simulink model "milemate_digital_twin"  (R2026a)
settings: Solver=VariableStepAuto  StopTime=500  MaxStep=0.05
libraries: sim3dlib x36
(part 4 of 5)

== matlab function milemate_digital_twin/MATLAB Function ==
  data: floor1_visual_id input size=[5 1]; floor1_visible input size=[50 1]; floor1_color_flag input size=[50 1]; platform_y input size=[1 1]; floor1_visual_count input size=[1 1]; pkg1_T output; pkg2_T output; pkg3_T output; pkg4_T output; pkg5_T output; pkg1_R output; pkg2_R output; pkg3_R output; pkg4_R output; pkg5_R output; pkg1_S output; pkg2_S output; pkg3_S output; pkg4_S output; pkg5_S output; target_unload_id input size=[1 1]; highlight_enable input size=[1 1]; target_package_on_belt4 input size=[1 1]; package_on_platform_from_floor input; platform_z input; current_unload_id input; floor1_visual_path input size=[5 1]; target_list input size=[20 1]; target_count input size=[1 1]; pkg1_Color output; pkg2_Color output; pkg3_Color output; pkg4_Color output; pkg5_Color output; belt4_reverse_progress input size=[1 1]; belt4_reverse_phase input size=[1 1]
function [pkg1_T, pkg2_T, pkg3_T, pkg4_T, pkg5_T, ...
          pkg1_R, pkg2_R, pkg3_R, pkg4_R, pkg5_R, ...
          pkg1_S, pkg2_S, pkg3_S, pkg4_S, pkg5_S, ...
          pkg1_Color, pkg2_Color, pkg3_Color, pkg4_Color, pkg5_Color] = ...
          Package3DMappingFunction_F1(floor1_visual_id, floor1_visible, floor1_color_flag, platform_y, floor1_visual_count, ...
                                      target_unload_id, highlight_enable, target_package_on_belt4, ...
                                      package_on_platform_from_floor, platform_z, current_unload_id, floor1_visual_path, ...
                                      target_list, target_count, belt4_reverse_progress, belt4_reverse_phase)
% Package3DMappingFunction_F1
% 1층 정적/연속 이동 박스 표시 함수
%
% 중요:
% - 이제 F1은 FloorStorageUpdate/floor1_queue 또는 PackageSlotVisualizer/floor1_slot_id를 직접 쓰지 않는다.
% - Floor1VisualStateFunction이 저장한 floor1_visual_id, floor1_visual_path를 기준으로 표시한다.
% - visual_shift는 이 함수에 직접 들어오지 않는다.
%
% 입력:
% floor1_visual_id               [5x1]
% floor1_visible                 [50x1]  % 기존 포트 유지용
% floor1_color_flag              [50x1]  % 기존 포트 유지용
% platform_y                     [1x1]
% floor1_visual_count            [1x1]
% target_unload_id               [1x1]  % 1층 하차공간 준비 대상
% highlight_enable               [1x1]
% target_package_on_belt4        [1x1]
% package_on_platform_from_floor [1x1]
% platform_z                     [1x1]
% current_unload_id              [1x1]  % 현재 실제 하차 대상
% floor1_visual_path             [5x1]

% =========================
% 박스 크기
% =========================
pkg_short = 0.12;
pkg_long  = 0.16;
pkg_h     = 0.08;

pkg_scale = [pkg_short, pkg_long, pkg_h];

% =========================
% 색상 설정
% =========================
normal_color = [0.75, 0.45, 0.20];
target_color = [1.0, 1.0, 0.0];

% =========================
% 1층 높이
% =========================
z_floor1 = 0.00;
pkg_center_z = z_floor1 + pkg_h / 2;

hide_z = -10.0;

% =========================
% 컨베이어 기준값
% =========================
belt_width = 0.25;

L1 = 0.51;
L3 = 0.51;
L4 = 1.11;

stopper_x = -0.15;
stopper_y = platform_y + 0.30;
stopper_thick_x = 0.03;

A_x = stopper_x - stopper_thick_x / 2;
A_y = stopper_y;

side_y = 1;
side_x = 1;

% =========================
% Belt3 geometry
% =========================
belt3_right_x = A_x;
belt3_center_y = A_y;
belt3_connect_edge_y = belt3_center_y + side_y * belt_width / 2;

% =========================
% Belt4 geometry
% =========================
if side_x > 0
    belt4_left_x  = A_x;
    belt4_right_x = A_x + belt_width;
else
    belt4_left_x  = A_x - belt_width;
    belt4_right_x = A_x;
end

belt4_center_x = (belt4_left_x + belt4_right_x) / 2;

belt4_start_y_nominal = belt3_connect_edge_y;
belt4_platform_extend = 0.25;

belt4_start_y = belt4_start_y_nominal - side_y * belt4_platform_extend;
belt4_end_y = belt4_start_y_nominal + side_y * L4;

if side_x > 0
    belt4_outer_x = belt4_right_x;
else
    belt4_outer_x = belt4_left_x;
end

% =========================
% 하차공간 좌표
% =========================
handoff_x = belt4_center_x;
handoff_y = belt4_start_y + side_y * (pkg_short / 2 + 0.02);
handoff_z = pkg_center_z;
handoff_yaw = pi / 2;

% Belt4 앞쪽 최대 위치 제한
belt4_max_y = belt4_end_y - side_y * (pkg_short / 2 + 0.02);

% =========================
% 플랫폼 위 회수 박스 좌표
% =========================
platform_pkg_x = 0.0;
platform_pkg_y = platform_y;
platform_pkg_z = platform_z + pkg_h / 2;
platform_pkg_yaw = pi / 2;

% =========================
% Belt1 geometry
% =========================
belt1_right_x = belt4_outer_x;
belt1_left_x  = belt1_right_x - L1;

belt1_inner_edge_y = belt4_end_y;
belt1_outer_edge_y = belt1_inner_edge_y + side_y * belt_width;

% =========================
% Belt2 geometry
% =========================
belt2_right_x = belt1_left_x;
belt2_left_x  = belt2_right_x - belt_width;
belt2_center_x = (belt2_left_x + belt2_right_x) / 2;

belt2_end_y = belt3_connect_edge_y;

% =========================
% 슬롯 배치 파라미터
% =========================
max_on_belt3 = 4;

pkg_visual_gap = 0.005;
slot_pitch = pkg_short + pkg_visual_gap;

stopper_center_gap = pkg_short / 2;
belt2_entry_gap = 0.04;

% =========================
% 기존 입력 포트 사용 처리
% =========================
% floor1_visible, floor1_color_flag는 기존 모델 연결을 유지하기 위한 입력이다.
% 현재 F1은 floor1_visual_id/path 기준으로 동작한다.
dummy_keep = floor1_visible(1) + floor1_color_flag(1);
dummy_keep = dummy_keep + 0;

% =========================
% 표시 여부
% =========================
visible1 = (floor1_visual_id(1) > 0);
visible2 = (floor1_visual_id(2) > 0);
visible3 = (floor1_visual_id(3) > 0);
visible4 = (floor1_visual_id(4) > 0);
visible5 = (floor1_visual_id(5) > 0);

% =========================
% 각 박스 생성
% =========================
[pkg1_T, pkg1_R, pkg1_S, pkg1_Color] = makePkg(floor1_visual_id(1), floor1_visual_path(1), visible1, ...
    belt3_right_x, belt3_center_y, belt2_center_x, belt2_end_y, ...
    belt4_center_x, belt4_max_y, ...
    slot_pitch, stopper_center_gap, belt2_entry_gap, max_on_belt3, ...
    pkg_center_z, hide_z, pkg_scale, side_y, ...
    target_unload_id, highlight_enable, target_package_on_belt4, ...
    handoff_x, handoff_y, handoff_z, handoff_yaw, ...
    package_on_platform_from_floor, platform_pkg_x, platform_pkg_y, platform_pkg_z, platform_pkg_yaw, ...
    current_unload_id, normal_color, target_color, target_list, target_count, belt4_reverse_progress, belt4_reverse_phase);

[pkg2_T, pkg2_R, pkg2_S, pkg2_Color] = makePkg(floor1_visual_id(2), floor1_visual_path(2), visible2, ...
    belt3_right_x, belt3_center_y, belt2_center_x, belt2_end_y, ...
    belt4_center_x, belt4_max_y, ...
    slot_pitch, stopper_center_gap, belt2_entry_gap, max_on_belt3, ...
    pkg_center_z, hide_z, pkg_scale, side_y, ...
    target_unload_id, highlight_enable, target_package_on_belt4, ...
    handoff_x, handoff_y, handoff_z, handoff_yaw, ...
    package_on_platform_from_floor, platform_pkg_x, platform_pkg_y, platform_pkg_z, platform_pkg_yaw, ...
    current_unload_id, normal_color, target_color, target_list, target_count, belt4_reverse_progress, belt4_reverse_phase);

[pkg3_T, pkg3_R, pkg3_S, pkg3_Color] = makePkg(floor1_visual_id(3), floor1_visual_path(3), visible3, ...
    belt3_right_x, belt3_center_y, belt2_center_x, belt2_end_y, ...
    belt4_center_x, belt4_max_y, ...
    slot_pitch, stopper_center_gap, belt2_entry_gap, max_on_belt3, ...
    pkg_center_z, hide_z, pkg_scale, side_y, ...
    target_unload_id, highlight_enable, target_package_on_belt4, ...
    handoff_x, handoff_y, handoff_z, handoff_yaw, ...
    package_on_platform_from_floor, platform_pkg_x, platform_pkg_y, platform_pkg_z, platform_pkg_yaw, ...
    current_unload_id, normal_color, target_color, target_list, target_count, belt4_reverse_progress, belt4_reverse_phase);

[pkg4_T, pkg4_R, pkg4_S, pkg4_Color] = makePkg(floor1_visual_id(4), floor1_visual_path(4), visible4, ...
    belt3_right_x, belt3_center_y, belt2_center_x, belt2_end_y, ...
    belt4_center_x, belt4_max_y, ...
    slot_pitch, stopper_center_gap, belt2_entry_gap, max_on_belt3, ...
    pkg_center_z, hide_z, pkg_scale, side_y, ...
    target_unload_id, highlight_enable, target_package_on_belt4, ...
    handoff_x, handoff_y, handoff_z, handoff_yaw, ...
    package_on_platform_from_floor, platform_pkg_x, platform_pkg_y, platform_pkg_z, platform_pkg_yaw, ...
    current_unload_id, normal_color, target_color, target_list, target_count, belt4_reverse_progress, belt4_reverse_phase);

[pkg5_T, pkg5_R, pkg5_S, pkg5_Color] = makePkg(floor1_visual_id(5), floor1_visual_path(5), visible5, ...
    belt3_right_x, belt3_center_y, belt2_center_x, belt2_end_y, ...
    belt4_center_x, belt4_max_y, ...
    slot_pitch, stopper_center_gap, belt2_entry_gap, max_on_belt3, ...
    pkg_center_z, hide_z, pkg_scale, side_y, ...
    target_unload_id, highlight_enable, target_package_on_belt4, ...
    handoff_x, handoff_y, handoff_z, handoff_yaw, ...
    package_on_platform_from_floor, platform_pkg_x, platform_pkg_y, platform_pkg_z, platform_pkg_yaw, ...
    current_unload_id, normal_color, target_color, target_list, target_count, belt4_reverse_progress, belt4_reverse_phase);

end


function [T, R, S, C] = makePkg(package_id, visual_path, visible, ...
                             belt3_right_x, belt3_y, ...
                             belt2_x, belt2_entry_y, ...
                             belt4_center_x, belt4_max_y, ...
                             slot_pitch, stopper_center_gap, belt2_entry_gap, ...
                             max_on_belt3, pkg_center_z, hide_z, pkg_scale, side_y, ...
                             target_unload_id, highlight_enable, target_package_on_belt4, ...
                             handoff_x, handoff_y, handoff_z, handoff_yaw, ...
                             package_on_platform_from_floor, platform_pkg_x, platform_pkg_y, platform_pkg_z, platform_pkg_yaw, ...
                             current_unload_id, normal_color, target_color, target_list, target_count, belt4_reverse_progress, belt4_reverse_phase)

C = normal_color;

% 상차 완료 후에만 target_list 안의 하차 대상 전체를 노란색으로 표시
if highlight_enable > 0.5
    if isUnloadTarget(package_id, target_list, target_count) > 0.5
        C = target_color;
    end
end

% 플랫폼 위에 올라간 현재 하차 대상도 노란색 유지
if package_on_platform_from_floor > 0.5 && package_id == current_unload_id && package_id > 0
    C = target_color;
end

if visible > 0.5 && package_id > 0

    % 1순위: Belt4 역회전으로 현재 하차대상 박스를 플랫폼까지 밀기
    % restore 중에는 이 조건을 타지 않고, 플랫폼 위에 고정되어야 한다.
    if belt4_reverse_phase == 1 && belt4_reverse_progress > 0 && package_id == current_unload_id && package_id > 0

        p = belt4_reverse_progress;

        if p < 0
            p = 0;
        end

        if p > 1
            p = 1;
        end

        push_to_x = platform_pkg_x;

        % 방향이 반대면 -를 +로 바꿔야 함
        push_to_y = handoff_y - side_y * 0.40;

        push_to_z = platform_pkg_z;

        x = handoff_x + p * (push_to_x - handoff_x);
        y = handoff_y + p * (push_to_y - handoff_y);
        z = handoff_z + p * (push_to_z - handoff_z);

        T = [x, y, z];
        R = [0, 0, platform_pkg_yaw];
        S = pkg_scale;
        C = target_color;
        return;
    end

    % 2순위: 플랫폼 위에 회수된 상태
    % 실제 현재 하차 대상만 플랫폼 위로 이동시킨다.
    if package_on_platform_from_floor > 0.5 && package_id == current_unload_id && package_id > 0
        T = [platform_pkg_x, platform_pkg_y, platform_pkg_z];
        R = [0, 0, platform_pkg_yaw];
        S = pkg_scale;
        return;
    end

    % 3순위: 시각화 상태에서 받은 visual_path 위치에 표시
    [x, y, yaw] = getContinuousPose(visual_path, ...
        belt3_right_x, belt3_y, ...
        belt2_x, belt2_entry_y, ...
        belt4_center_x, belt4_max_y, ...
        slot_pitch, stopper_center_gap, belt2_entry_gap, ...
        max_on_belt3, side_y, ...
        handoff_x, handoff_y, handoff_yaw);

    T = [x, y, pkg_center_z];
    R = [0, 0, yaw];
    S = pkg_scale;

else
    T = [0, 0, hide_z];
    R = [0, 0, 0];
    S = pkg_scale;
end

end


function [x, y, yaw] = getContinuousPose(path_pos, ...
                                         belt3_right_x, belt3_y, ...
                                         belt2_x, belt2_entry_y, ...
                                         belt4_center_x, belt4_max_y, ...
                                         slot_pitch, stopper_center_gap, belt2_entry_gap, ...
                                         max_on_belt3, side_y, ...
                                         handoff_x, handoff_y, handoff_yaw)
% getContinuousPose
%
% path_pos 기준:
% path_pos = 4 : 기존 slot4 위치
% path_pos = 3 : 기존 slot3 위치
% path_pos = 2 : 기존 slot2 위치
% path_pos = 1 : 기존 slot1 위치
% path_pos = 0 : 하차공간
% path_pos < 0 : 하차공간보다 앞쪽 Belt4 위

upper_idx = ceil(path_pos);
lower_idx = floor(path_pos);

if upper_idx == lower_idx
    [x, y, yaw] = getIntegerPose(upper_idx, ...
        belt3_right_x, belt3_y, ...
        belt2_x, belt2_entry_y, ...
        belt4_center_x, belt4_max_y, ...
        slot_pitch, stopper_center_gap, belt2_entry_gap, ...
        max_on_belt3, side_y, ...
        handoff_x, handoff_y, handoff_yaw);
else
    alpha = upper_idx - path_pos;

    if alpha < 0
        alpha = 0;
    end

    if alpha > 1
        alpha = 1;
    end

    [x_upper, y_upper, yaw_upper] = getIntegerPose(upper_idx, ...
        belt3_right_x, belt3_y, ...
        belt2_x, belt2_entry_y, ...
        belt4_center_x, belt4_max_y, ...
        slot_pitch, stopper_center_gap, belt2_entry_gap, ...
        max_on_belt3, side_y, ...
        handoff_x, handoff_y, handoff_yaw);

    [x_lower, y_lower, yaw_lower] = getIntegerPose(lower_idx, ...
        belt3_right_x, belt3_y, ...
        belt2_x, belt2_entry_y, ...
        belt4_center_x, belt4_max_y, ...
        slot_pitch, stopper_center_gap, belt2_entry_gap, ...
        max_on_belt3, side_y, ...
        handoff_x, handoff_y, handoff_yaw);

    x = x_upper + alpha * (x_lower - x_upper);
    y = y_upper + alpha * (y_lower - y_upper);

    if alpha < 0.5
        yaw = yaw_upper;
    else
        yaw = yaw_lower;
    end
end

end


function [x, y, yaw] = getIntegerPose(idx, ...
                                      belt3_right_x, belt3_y, ...
                                      belt2_x, belt2_entry_y, ...
                                      belt4_center_x, belt4_max_y, ...
                                      slot_pitch, stopper_center_gap, belt2_entry_gap, ...
                                      max_on_belt3, side_y, ...
                                      handoff_x, handoff_y, handoff_yaw)
% getIntegerPose
%
% idx >= 1:
%   기존 Belt3/Belt2 슬롯 위치
%
% idx == 0:
%   하차공간
%
% idx < 0:
%   하차공간보다 더 앞쪽의 Belt4 위치

if idx <= 0

    x = belt4_center_x;
    y = handoff_y + side_y * (-idx) * slot_pitch;

    if side_y > 0
        if y > belt4_max_y
            y = belt4_max_y;
        end
    else
        if y < belt4_max_y
            y = belt4_max_y;
        end
    end

    yaw = handoff_yaw;

elseif idx <= max_on_belt3

    d = stopper_center_gap + slot_pitch * (idx - 1);

    x = belt3_right_x - d;
    y = belt3_y;

    yaw = 0;

else

    k = idx - max_on_belt3;

    x = belt2_x;
    y = belt2_entry_y + side_y * (belt2_entry_gap + slot_pitch * (k - 1));

    yaw = pi / 2;

end

end

function flag = isUnloadTarget(package_id, target_list, target_count)
% target_list에 package_id가 있으면 1, 아니면 0

flag = 0;

if package_id <= 0
    return;
end

n = target_count;

if n < 0
    n = 0;
end

if n > 20
    n = 20;
end

for i = 1:20
    if i <= n
        if target_list(i) == package_id
            flag = 1;
        end
    end
end

end

== matlab function milemate_digital_twin/MATLAB Function1 ==
  data: floor3_visual_id input size=[6 1]; floor3_visible input size=[50 1]; floor3_color_flag input size=[50 1]; platform_y input size=[1 1]; floor3_visual_count input; pkg1_T output; pkg2_T output; pkg3_T output; pkg4_T output; pkg5_T output; pkg6_T output; pkg1_R output; pkg2_R output; pkg3_R output; pkg4_R output; pkg5_R output; pkg6_R output; pkg1_S output; pkg2_S output; pkg3_S output; pkg4_S output; pkg5_S output; target_unload_id input size=[1 1]; highlight_enable input size=[1 1]; target_package_on_belt4 input size=[1 1]; pkg6_S output; package_on_platform_from_floor input; platform_z input; current_unload_id input; floor3_visual_path input size=[6 1]; target_list input size=[20 1]; target_count input size=[1 1]; pkg1_Color output; pkg2_Color output; pkg3_Color output; pkg4_Color output; pkg5_Color output; pkg6_Color output; belt4_reverse_progress input; belt4_reverse_phase input
function [pkg1_T, pkg2_T, pkg3_T, pkg4_T, pkg5_T, pkg6_T, ...
          pkg1_R, pkg2_R, pkg3_R, pkg4_R, pkg5_R, pkg6_R, ...
          pkg1_S, pkg2_S, pkg3_S, pkg4_S, pkg5_S, pkg6_S, ...
          pkg1_Color, pkg2_Color, pkg3_Color, pkg4_Color, pkg5_Color, pkg6_Color] = ...
          Package3DMappingFunction_F3(floor3_visual_id, floor3_visible, floor3_color_flag, platform_y, floor3_visual_count, ...
                                      target_unload_id, highlight_enable, target_package_on_belt4, ...
                                      package_on_platform_from_floor, platform_z, current_unload_id, floor3_visual_path, ...
                                      target_list, target_count, belt4_reverse_progress, belt4_reverse_phase)
% Package3DMappingFunction_F3
% 3층 정적/연속 이동 박스 표시 함수
%
% 중요:
% - 이제 F3는 FloorStorageUpdate/floor3_queue 또는 PackageSlotVisualizer/floor3_slot_id를 직접 쓰지 않는다.
% - Floor3VisualStateFunction이 저장한 floor3_visual_id, floor3_visual_path를 기준으로 표시한다.
% - visual_shift는 이 함수에 직접 들어오지 않는다.
%
% 입력:
% floor3_visual_id               [6x1]
% floor3_visible                 [50x1]  % 기존 포트 유지용
% floor3_color_flag              [50x1]  % 기존 포트 유지용
% platform_y                     [1x1]
% floor3_visual_count            [1x1]
% target_unload_id               [1x1]
% highlight_enable               [1x1]
% target_package_on_belt4        [1x1]
% package_on_platform_from_floor [1x1]
% platform_z                     [1x1]
% current_unload_id              [1x1]
% floor3_visual_path             [6x1]
% target_list                    [20x1]
% target_count                   [1x1]

% =========================
% 박스 크기
% =========================
pkg_short = 0.12;
pkg_long  = 0.16;
pkg_h     = 0.08;

pkg_scale = [pkg_short, pkg_long, pkg_h];

% =========================
% 색상 설정
% =========================
% Actor 기본 색이 갈색이면 normal_color는 흰색으로 둔다.
normal_color = [0.75, 0.45, 0.20];
target_color = [1.0, 1.0, 0.0];

% =========================
% 3층 높이
% =========================
z_floor3 = 0.54;
pkg_center_z = z_floor3 + pkg_h / 2;

hide_z = -10.0;

% =========================
% 컨베이어 기준값
% =========================
belt_width = 0.25;

L1 = 0.51;
L3 = 0.51;
L4 = 1.11;

stopper_x = -0.15;
stopper_y = platform_y + 0.30;
stopper_thick_x = 0.03;

A_x = stopper_x - stopper_thick_x / 2;
A_y = stopper_y;

side_y = 1;
side_x = 1;

% =========================
% Belt3 geometry
% =========================
belt3_right_x = A_x;
belt3_center_y = A_y;
belt3_connect_edge_y = belt3_center_y + side_y * belt_width / 2;

% =========================
% Belt4 geometry
% =========================
if side_x > 0
    belt4_left_x  = A_x;
    belt4_right_x = A_x + belt_width;
else
    belt4_left_x  = A_x - belt_width;
    belt4_right_x = A_x;
end

belt4_center_x = (belt4_left_x + belt4_right_x) / 2;

belt4_start_y_nominal = belt3_connect_edge_y;
belt4_platform_extend = 0.25;

belt4_start_y = belt4_start_y_nominal - side_y * belt4_platform_extend;
belt4_end_y = belt4_start_y_nominal + side_y * L4;

if side_x > 0
    belt4_outer_x = belt4_right_x;
else
    belt4_outer_x = belt4_left_x;
end

% =========================
% 하차공간 좌표
% =========================
handoff_x = belt4_center_x;
handoff_y = belt4_start_y + side_y * (pkg_short / 2 + 0.02);
handoff_z = pkg_center_z;
handoff_yaw = pi / 2;

% Belt4 앞쪽 최대 위치 제한
belt4_max_y = belt4_end_y - side_y * (pkg_short / 2 + 0.02);

% =========================
% 플랫폼 위 회수 박스 좌표
% =========================
platform_pkg_x = 0.0;
platform_pkg_y = platform_y;
platform_pkg_z = platform_z + pkg_h / 2;
platform_pkg_yaw = pi / 2;

% =========================
% Belt1 geometry
% =========================
belt1_right_x = belt4_outer_x;
belt1_left_x  = belt1_right_x - L1;

belt1_inner_edge_y = belt4_end_y;
belt1_outer_edge_y = belt1_inner_edge_y + side_y * belt_width;

% =========================
% Belt2 geometry
% =========================
belt2_right_x = belt1_left_x;
belt2_left_x  = belt2_right_x - belt_width;
belt2_center_x = (belt2_left_x + belt2_right_x) / 2;

belt2_end_y = belt3_connect_edge_y;

% =========================
% 슬롯 배치 파라미터
% =========================
max_on_belt3 = 4;

pkg_visual_gap = 0.005;
slot_pitch = pkg_short + pkg_visual_gap;

stopper_center_gap = pkg_short / 2;
belt2_entry_gap = 0.04;

% =========================
% 기존 입력 포트 사용 처리
% =========================
dummy_keep = floor3_visible(1) + floor3_color_flag(1);
dummy_keep = dummy_keep + 0;

% =========================
% 표시 여부
% =========================
% visual state는 중간 빈칸을 허용하므로 count 기준으로 visible을 판단하면 안 된다.
visible1 = (floor3_visual_id(1) > 0);
visible2 = (floor3_visual_id(2) > 0);
visible3 = (floor3_visual_id(3) > 0);
visible4 = (floor3_visual_id(4) > 0);
visible5 = (floor3_visual_id(5) > 0);
visible6 = (floor3_visual_id(6) > 0);

% =========================
% 각 박스 생성
% =========================
[pkg1_T, pkg1_R, pkg1_S, pkg1_Color] = makePkg(floor3_visual_id(1), floor3_visual_path(1), visible1, ...
    belt3_right_x, belt3_center_y, belt2_center_x, belt2_end_y, ...
    belt4_center_x, belt4_max_y, ...
    slot_pitch, stopper_center_gap, belt2_entry_gap, max_on_belt3, ...
    pkg_center_z, hide_z, pkg_scale, side_y, ...
    target_unload_id, highlight_enable, target_package_on_belt4, ...
    handoff_x, handoff_y, handoff_z, handoff_yaw, ...
    package_on_platform_from_floor, platform_pkg_x, platform_pkg_y, platform_pkg_z, platform_pkg_yaw, ...
    current_unload_id, normal_color, target_color, target_list, target_count, belt4_reverse_progress, belt4_reverse_phase);

[pkg2_T, pkg2_R, pkg2_S, pkg2_Color] = makePkg(floor3_visual_id(2), floor3_visual_path(2), visible2, ...
    belt3_right_x, belt3_center_y, belt2_center_x, belt2_end_y, ...
    belt4_center_x, belt4_max_y, ...
    slot_pitch, stopper_center_gap, belt2_entry_gap, max_on_belt3, ...
    pkg_center_z, hide_z, pkg_scale, side_y, ...
    target_unload_id, highlight_enable, target_package_on_belt4, ...
    handoff_x, handoff_y, handoff_z, handoff_yaw, ...
    package_on_platform_from_floor, platform_pkg_x, platform_pkg_y, platform_pkg_z, platform_pkg_yaw, ...
    current_unload_id, normal_color, target_color, target_list, target_count, belt4_reverse_progress, belt4_reverse_phase);

[pkg3_T, pkg3_R, pkg3_S, pkg3_Color] = makePkg(floor3_visual_id(3), floor3_visual_path(3), visible3, ...
    belt3_right_x, belt3_center_y, belt2_center_x, belt2_end_y, ...
    belt4_center_x, belt4_max_y, ...
    slot_pitch, stopper_center_gap, belt2_entry_gap, max_on_belt3, ...
    pkg_center_z, hide_z, pkg_scale, side_y, ...
    target_unload_id, highlight_enable, target_package_on_belt4, ...
    handoff_x, handoff_y, handoff_z, handoff_yaw, ...
    package_on_platform_from_floor, platform_pkg_x, platform_pkg_y, platform_pkg_z, platform_pkg_yaw, ...
    current_unload_id, normal_color, target_color, target_list, target_count, belt4_reverse_progress, belt4_reverse_phase);

[pkg4_T, pkg4_R, pkg4_S, pkg4_Color] = makePkg(floor3_visual_id(4), floor3_visual_path(4), visible4, ...
    belt3_right_x, belt3_center_y, belt2_center_x, belt2_end_y, ...
    belt4_center_x, belt4_max_y, ...
    slot_pitch, stopper_center_gap, belt2_entry_gap, max_on_belt3, ...
    pkg_center_z, hide_z, pkg_scale, side_y, ...
    target_unload_id, highlight_enable, target_package_on_belt4, ...
    handoff_x, handoff_y, handoff_z, handoff_yaw, ...
    package_on_platform_from_floor, platform_pkg_x, platform_pkg_y, platform_pkg_z, platform_pkg_yaw, ...
    current_unload_id, normal_color, target_color, target_list, target_count, belt4_reverse_progress, belt4_reverse_phase);

[pkg5_T, pkg5_R, pkg5_S, pkg5_Color] = makePkg(floor3_visual_id(5), floor3_visual_path(5), visible5, ...
    belt3_right_x, belt3_center_y, belt2_center_x, belt2_end_y, ...
    belt4_center_x, belt4_max_y, ...
    slot_pitch, stopper_center_gap, belt2_entry_gap, max_on_belt3, ...
    pkg_center_z, hide_z, pkg_scale, side_y, ...
    target_unload_id, highlight_enable, target_package_on_belt4, ...
    handoff_x, handoff_y, handoff_z, handoff_yaw, ...
    package_on_platform_from_floor, platform_pkg_x, platform_pkg_y, platform_pkg_z, platform_pkg_yaw, ...
    current_unload_id, normal_color, target_color, target_list, target_count, belt4_reverse_progress, belt4_reverse_phase);

[pkg6_T, pkg6_R, pkg6_S, pkg6_Color] = makePkg(floor3_visual_id(6), floor3_visual_path(6), visible6, ...
    belt3_right_x, belt3_center_y, belt2_center_x, belt2_end_y, ...
    belt4_center_x, belt4_max_y, ...
    slot_pitch, stopper_center_gap, belt2_entry_gap, max_on_belt3, ...
    pkg_center_z, hide_z, pkg_scale, side_y, ...
    target_unload_id, highlight_enable, target_package_on_belt4, ...
    handoff_x, handoff_y, handoff_z, handoff_yaw, ...
    package_on_platform_from_floor, platform_pkg_x, platform_pkg_y, platform_pkg_z, platform_pkg_yaw, ...
    current_unload_id, normal_color, target_color, target_list, target_count, belt4_reverse_progress, belt4_reverse_phase);

end


function [T, R, S, C] = makePkg(package_id, visual_path, visible, ...
                                 belt3_right_x, belt3_y, ...
                                 belt2_x, belt2_entry_y, ...
                                 belt4_center_x, belt4_max_y, ...
                                 slot_pitch, stopper_center_gap, belt2_entry_gap, ...
                                 max_on_belt3, pkg_center_z, hide_z, pkg_scale, side_y, ...
                                 target_unload_id, highlight_enable, target_package_on_belt4, ...
                                 handoff_x, handoff_y, handoff_z, handoff_yaw, ...
                                 package_on_platform_from_floor, platform_pkg_x, platform_pkg_y, platform_pkg_z, platform_pkg_yaw, ...
                                 current_unload_id, normal_color, target_color, target_list, target_count, belt4_reverse_progress, belt4_reverse_phase)

C = normal_color;

% 상차 완료 후에만 target_list 안의 하차 대상 전체를 노란색으로 표시
if highlight_enable > 0.5
    if isUnloadTarget(package_id, target_list, target_count) > 0.5
        C = target_color;
    end
end

% 플랫폼 위에 올라간 현재 하차 대상도 노란색 유지
if package_on_platform_from_floor > 0.5 && package_id == current_unload_id && package_id > 0
    C = target_color;
end

if visible > 0.5 && package_id > 0

    % 1순위: Belt4 역회전으로 현재 하차대상 박스를 플랫폼까지 밀기
    % restore 중에는 이 조건을 타지 않고, 플랫폼 위에 고정되어야 한다.
    if belt4_reverse_phase == 1 && belt4_reverse_progress > 0 && package_id == current_unload_id && package_id > 0

        p = belt4_reverse_progress;

        if p < 0
            p = 0;
        end

        if p > 1
            p = 1;
        end

        push_to_x = platform_pkg_x;

        % 방향이 반대면 -를 +로 바꿔야 함
        push_to_y = handoff_y - side_y * 0.40;

        push_to_z = platform_pkg_z;

        x = handoff_x + p * (push_to_x - handoff_x);
        y = handoff_y + p * (push_to_y - handoff_y);
        z = handoff_z + p * (push_to_z - handoff_z);

        T = [x, y, z];
        R = [0, 0, platform_pkg_yaw];
        S = pkg_scale;
        C = target_color;
        return;
    end

    % 2순위: 플랫폼 위에 회수된 상태
    if package_on_platform_from_floor > 0.5 && package_id == current_unload_id && package_id > 0
        T = [platform_pkg_x, platform_pkg_y, platform_pkg_z];
        R = [0, 0, platform_pkg_yaw];
        S = pkg_scale;
        return;
    end

    % 3순위: visual_path 위치 표시
    [x, y, yaw] = getContinuousPose(visual_path, ...
        belt3_right_x, belt3_y, ...
        belt2_x, belt2_entry_y, ...
        belt4_center_x, belt4_max_y, ...
        slot_pitch, stopper_center_gap, belt2_entry_gap, ...
        max_on_belt3, side_y, ...
        handoff_x, handoff_y, handoff_yaw);

    T = [x, y, pkg_center_z];
    R = [0, 0, yaw];
    S = pkg_scale;

else
    T = [0, 0, hide_z];
    R = [0, 0, 0];
    S = pkg_scale;
end

end


function [x, y, yaw] = getContinuousPose(path_pos, ...
                                         belt3_right_x, belt3_y, ...
                                         belt2_x, belt2_entry_y, ...
                                         belt4_center_x, belt4_max_y, ...
                                         slot_pitch, stopper_center_gap, belt2_entry_gap, ...
                                         max_on_belt3, side_y, ...
                                         handoff_x, handoff_y, handoff_yaw)

upper_idx = ceil(path_pos);
lower_idx = floor(path_pos);

if upper_idx == lower_idx
    [x, y, yaw] = getIntegerPose(upper_idx, ...
        belt3_right_x, belt3_y, ...
        belt2_x, belt2_entry_y, ...
        belt4_center_x, belt4_max_y, ...
        slot_pitch, stopper_center_gap, belt2_entry_gap, ...
        max_on_belt3, side_y, ...
        handoff_x, handoff_y, handoff_yaw);
else
    alpha = upper_idx - path_pos;

    if alpha < 0
        alpha = 0;
    end

    if alpha > 1
        alpha = 1;
    end

    [x_upper, y_upper, yaw_upper] = getIntegerPose(upper_idx, ...
        belt3_right_x, belt3_y, ...
        belt2_x, belt2_entry_y, ...
        belt4_center_x, belt4_max_y, ...
        slot_pitch, stopper_center_gap, belt2_entry_gap, ...
        max_on_belt3, side_y, ...
        handoff_x, handoff_y, handoff_yaw);

    [x_lower, y_lower, yaw_lower] = getIntegerPose(lower_idx, ...
        belt3_right_x, belt3_y, ...
        belt2_x, belt2_entry_y, ...
        belt4_center_x, belt4_max_y, ...
        slot_pitch, stopper_center_gap, belt2_entry_gap, ...
        max_on_belt3, side_y, ...
        handoff_x, handoff_y, handoff_yaw);

    x = x_upper + alpha * (x_lower - x_upper);
    y = y_upper + alpha * (y_lower - y_upper);

    if alpha < 0.5
        yaw = yaw_upper;
    else
        yaw = yaw_lower;
    end
end

end


function [x, y, yaw] = getIntegerPose(idx, ...
                                      belt3_right_x, belt3_y, ...
                                      belt2_x, belt2_entry_y, ...
                                      belt4_center_x, belt4_max_y, ...
                                      slot_pitch, stopper_center_gap, belt2_entry_gap, ...
                                      max_on_belt3, side_y, ...
                                      handoff_x, handoff_y, handoff_yaw)

if idx <= 0

    x = belt4_center_x;
    y = handoff_y + side_y * (-idx) * slot_pitch;

    if side_y > 0
        if y > belt4_max_y
            y = belt4_max_y;
        end
    else
        if y < belt4_max_y
            y = belt4_max_y;
        end
    end

    yaw = handoff_yaw;

elseif idx <= max_on_belt3

    d = stopper_center_gap + slot_pitch * (idx - 1);

    x = belt3_right_x - d;
    y = belt3_y;

    yaw = 0;

else

    k = idx - max_on_belt3;

    x = belt2_x;
    y = belt2_entry_y + side_y * (belt2_entry_gap + slot_pitch * (k - 1));

    yaw = pi / 2;

end

end


function flag = isUnloadTarget(package_id, target_list, target_count)
flag = 0;

if package_id <= 0
    return;
end

n = target_count;

if n < 0
    n = 0;
end

if n > 20
    n = 20;
end

for i = 1:20
    if i <= n
        if target_list(i) == package_id
            flag = 1;
        end
    end
end

end

== matlab function milemate_digital_twin/MATLAB Function3 ==
  data: moving_arrive_done input; visual_count_f1 output; moving_arrive_floor input; visual_count_f2 output; visual_count_f3 output; visual_count_selected output; current_target_floor input
function [visual_count_f1, visual_count_f2, visual_count_f3, visual_count_selected] = ...
    FloorVisualArrivalCounterFunction(moving_arrive_done, moving_arrive_floor, current_target_floor)
% FloorVisualArrivalCounterFunction
%
% 목적:
% - MovingPackage가 실제 도착했을 때 층별 visual_count 증가
% - moving_arrive_done 펄스를 기준으로 카운트
% - moving_arrive_floor가 정상값(1,2,3)이면 그 값을 사용
% - moving_arrive_floor가 0이면 current_target_floor를 fallback으로 사용
%
% 입력:
% moving_arrive_done   : MovingPackage 도착 펄스
% moving_arrive_floor  : MovingPackage가 latch한 도착 층
% current_target_floor : 현재 목표층
%
% 출력:
% visual_count_f1
% visual_count_f2
% visual_count_f3
% visual_count_selected

persistent count_f1 count_f2 count_f3 prev_arrive

if isempty(count_f1)
    count_f1 = 0;
    count_f2 = 0;
    count_f3 = 0;
    prev_arrive = 0;
end

arrive_now = moving_arrive_done > 0.5;
arrive_rising = arrive_now && (prev_arrive <= 0.5);

if arrive_rising

    % 우선 MovingPackage가 알려준 도착 층을 사용
    arrived_floor = moving_arrive_floor;

    % moving_arrive_floor가 0 또는 비정상값이면 현재 target_floor로 대체
    if arrived_floor < 1 || arrived_floor > 3
        arrived_floor = current_target_floor;
    end

    if arrived_floor == 1
        count_f1 = count_f1 + 1;

    elseif arrived_floor == 2
        count_f2 = count_f2 + 1;

    elseif arrived_floor == 3
        count_f3 = count_f3 + 1;
    end
end

prev_arrive = double(arrive_now);

visual_count_f1 = count_f1;
visual_count_f2 = count_f2;
visual_count_f3 = count_f3;

if current_target_floor == 1
    visual_count_selected = count_f1;
elseif current_target_floor == 2
    visual_count_selected = count_f2;
elseif current_target_floor == 3
    visual_count_selected = count_f3;
else
    visual_count_selected = 0;
end

end

== matlab function milemate_digital_twin/UnloadTargetManager ==
  data: target_list input size=[20 1]; target_package_id output size=[1 1]; target_count input size=[1 1]; unload_done input size=[1 1]; mission_phase input size=[1 1]; current_target_index output size=[1 1]; unload_all_done output size=[1 1]
function [target_package_id, current_target_index, unload_all_done] = ...
    UnloadTargetManager(target_list, target_count, unload_done, mission_phase)
% UnloadTargetManager
%
% 목적:
% - 여러 개의 하차 대상 package_id를 순차적으로 선택한다.
% - unload_done이 발생하면 다음 하차 대상으로 넘어간다.
% - 모든 대상 하차가 끝나면 unload_all_done = 1을 출력한다.
%
% 입력:
% target_list   : 하차 대상 package_id 목록, 예: [4; 7; 0; 0; ...]
% target_count  : 실제 하차할 개수
% unload_done   : UnloadController의 하차 완료 신호
% mission_phase : MissionModeFunction의 현재 단계
%
% 출력:
% target_package_id     : 현재 하차 대상 package_id
% current_target_index  : 현재 몇 번째 하차 대상인지
% unload_all_done       : 모든 하차 대상 완료 여부

persistent idx
persistent prev_unload_done

MAX_TARGETS = 20;

if isempty(idx)
    idx = int32(1);
    prev_unload_done = 0;
end

% 기본 출력
target_package_id = 0;
current_target_index = double(idx);
unload_all_done = 0;

% target_count 정리
count = int32(target_count);

if count < 0
    count = int32(0);
end

if count > MAX_TARGETS
    count = int32(MAX_TARGETS);
end

% 하차 단계가 아니면 첫 번째 대상으로 대기
if mission_phase < 1
    idx = int32(1);
    prev_unload_done = unload_done;

    if count >= 1
        target_package_id = target_list(1);
    else
        target_package_id = 0;
    end

    current_target_index = double(idx);
    unload_all_done = 0;
    return;
end

% 하차할 대상이 없으면 완료
if count == 0
    target_package_id = 0;
    current_target_index = 0;
    unload_all_done = 1;
    prev_unload_done = unload_done;
    return;
end

% idx 범위 보정
if idx < 1
    idx = int32(1);
end

if idx > count
    target_package_id = 0;
    current_target_index = double(idx);
    unload_all_done = 1;
    prev_unload_done = unload_done;
    return;
end

% 현재 target 출력
% 중요:
% unload_done이 같은 step에 들어와도 이 step에서는 아직 현재 target을 출력한다.
% 그래야 FloorStorageUpdate가 현재 target을 보고 정확히 삭제할 수 있다.
target_package_id = target_list(idx);
current_target_index = double(idx);
unload_all_done = 0;

% unload_done 상승 에지 감지
unload_rising = (prev_unload_done == 0) && (unload_done == 1);

% 하차 완료되면 다음 step부터 다음 target으로 넘어가도록 idx 증가
if unload_rising
    idx = idx + 1;

    if idx > count
        unload_all_done = 1;
    end
end

prev_unload_done = unload_done;

end

== matlab function milemate_digital_twin/PlatformFoldControlFunction ==
  data: mission_phase input; platform_fold_angle output; delivery_arrived input; platform_deployed output; platform_z input
function [platform_fold_angle, platform_deployed] = PlatformFoldControlFunction(mission_phase, delivery_arrived, platform_z)
% PlatformFoldControlFunction
%
% 플랫폼 바닥판 접힘/펼침 각도를 부드럽게 생성한다.
%
% 입력:
% mission_phase:
%   0 = 상차
%   1 = 하차 준비/하차
%   2 = 미션 완료
%
% delivery_arrived:
%   0 = 배송 중 / 하차 준비
%   1 = 배달 장소 도착 / 실제 하차 가능
%
% platform_z:
%   현재 플랫폼 높이
%
% 출력:
% platform_fold_angle:
%   0    = 펼쳐진 상태
%   pi/2 = 접힌 상태
%
% platform_deployed:
%   1 = 거의 완전히 펼쳐짐
%   0 = 접힘 또는 접히는/펼쳐지는 중
%
% 핵심 규칙:
% - 상차 중에는 펼침
% - 배송 중 하차 준비 단계에서는 플랫폼이 1층에 도착한 뒤 접힘
% - 배송 중이라도 플랫폼이 1층이 아니면 접히지 않고 펼친 상태 유지
% - 배달 장소 도착 후 실제 하차 단계에서는 펼침
% - 미션 완료 후에는 1층에서 접힘

persistent angle

if isempty(angle)
    angle = pi/2;   % 시작은 접힌 상태
end

% =========================
% 1층 도착 판단
% =========================
floor1_z = 0.00;
floor_tol = 0.005;

platform_at_floor1 = 0;

if platform_z >= floor1_z - floor_tol && platform_z <= floor1_z + floor_tol
    platform_at_floor1 = 1;
end

% =========================
% 펼침/접힘 명령 판단
% =========================
% deploy_cmd = 1 → 펼침
% deploy_cmd = 0 → 접힘
deploy_cmd = 0;

% 상차 단계: 택배를 플랫폼 위에 올려야 하므로 펼침
if mission_phase == 0
    deploy_cmd = 1;
end

% 하차 준비/하차 단계
if mission_phase == 1

    if delivery_arrived > 0.5
        % 배달 장소 도착 후 실제 하차 단계는 펼침
        deploy_cmd = 1;
    else
        % 배송 중 하차 준비 단계
        % 플랫폼은 1층에 있으면 접고,
        % 1층이 아니면 먼저 1층 복귀 중이므로 펼친 상태 유지
        if platform_at_floor1 > 0.5
            deploy_cmd = 0;
        else
            deploy_cmd = 1;
        end
    end
end

% 미션 완료 후
if mission_phase >= 2
    if platform_at_floor1 > 0.5
        deploy_cmd = 0;
    else
        deploy_cmd = 1;
    end
end

% =========================
% 부드러운 각도 이동
% =========================
% 샘플타임 0.05 기준
% 0.04 rad/step이면 약 2초 정도에 90도 접힘/펼침
fold_step = 0.04;

if deploy_cmd > 0.5
    % 펼치기: pi/2 → 0
    angle = angle - fold_step;

    if angle < 0
        angle = 0;
    end
else
    % 접기: 0 → pi/2
    angle = angle + fold_step;

    if angle > pi/2
        angle = pi/2;
    end
end

platform_fold_angle = angle;

% 거의 완전히 펼쳐진 경우만 deployed = 1
if angle < 0.05
    platform_deployed = 1;
else
    platform_deployed = 0;
end

end

== matlab function milemate_digital_twin/FloorUnloadTargetSelector ==
  data: target_list input size=[20 1]; target_id_f1 output size=[1 1]; target_index_f1 output size=[1 1]; target_count input; floor1_queue input size=[50 1]; floor2_queue input size=[50 1]; floor3_queue input size=[50 1]; found_f1 output size=[1 1]; target_id_f2 output size=[1 1]; target_index_f2 output size=[1 1]; found_f2 output size=[1 1]; target_id_f3 output size=[1 1]; target_index_f3 output size=[1 1]; found_f3 output size=[1 1]
function [target_id_f1, target_index_f1, found_f1, ...
          target_id_f2, target_index_f2, found_f2, ...
          target_id_f3, target_index_f3, found_f3] = ...
          FloorUnloadTargetSelector(target_list, target_count, floor1_queue, floor2_queue, floor3_queue)
% FloorUnloadTargetSelector
%
% 목적:
% - 전체 하차 대상 리스트(target_list)를 보고,
%   각 층에서 먼저 준비해야 할 하차 대상 package_id와 queue index를 찾는다.
%
% 핵심 개념:
% - 하차 준비는 층별로 독립 가능하다.
% - 각 층 컨베이어는 개별로 움직일 수 있으므로,
%   1층, 2층, 3층 각각 하나의 하차 대상은 동시에 하차공간으로 미리 보낼 수 있다.
% - 단, 같은 층에 하차 대상이 여러 개 있으면 그 층에서는 target_list 순서상 가장 앞선 것 하나만 선택한다.
%
% 입력:
% target_list   [20x1] : 하차 대상 package_id 목록
% target_count  [1x1]  : 실제 하차 대상 개수
% floor1_queue  [50x1] : 1층 적재 queue
% floor2_queue  [50x1] : 2층 적재 queue
% floor3_queue  [50x1] : 3층 적재 queue
%
% 출력:
% target_id_fN     : 해당 층에서 먼저 준비할 package_id
% target_index_fN  : 해당 package_id가 현재 floorN_queue에서 몇 번째인지
% found_fN         : 해당 층에 준비 대상이 있으면 1, 없으면 0

MAX_TARGETS = 20;
QUEUE_MAX = 50;

% =========================
% 기본 출력
% =========================
target_id_f1 = 0;
target_index_f1 = 0;
found_f1 = 0;

target_id_f2 = 0;
target_index_f2 = 0;
found_f2 = 0;

target_id_f3 = 0;
target_index_f3 = 0;
found_f3 = 0;

% =========================
% target_count 보정
% =========================
count = int32(target_count);

if count < 0
    count = int32(0);
end

if count > MAX_TARGETS
    count = int32(MAX_TARGETS);
end

if count == 0
    return;
end

% =========================
% target_list 순서대로 탐색
% =========================
for t = 1:count
    target_id = target_list(t);

    if target_id <= 0
        continue;
    end

    % -------------------------
    % 1층 탐색
    % -------------------------
    if found_f1 < 0.5
        idx1 = findPackageIndex(floor1_queue, target_id, QUEUE_MAX);

        if idx1 > 0
            target_id_f1 = target_id;
            target_index_f1 = idx1;
            found_f1 = 1;
        end
    end

    % -------------------------
    % 2층 탐색
    % -------------------------
    if found_f2 < 0.5
        idx2 = findPackageIndex(floor2_queue, target_id, QUEUE_MAX);

        if idx2 > 0
            target_id_f2 = target_id;
            target_index_f2 = idx2;
            found_f2 = 1;
        end
    end

    % -------------------------
    % 3층 탐색
    % -------------------------
    if found_f3 < 0.5
        idx3 = findPackageIndex(floor3_queue, target_id, QUEUE_MAX);

        if idx3 > 0
            target_id_f3 = target_id;
            target_index_f3 = idx3;
            found_f3 = 1;
        end
    end

    % 세 층 모두 준비 대상이 정해졌으면 더 볼 필요 없음
    if found_f1 > 0.5 && found_f2 > 0.5 && found_f3 > 0.5
        break;
    end
end

end


function idx = findPackageIndex(queue, target_id, queue_max)
% queue 안에서 target_id의 위치를 찾는다.
% 없으면 0 반환.

idx = 0;

for i = 1:queue_max
    if queue(i) == target_id
        idx = i;
        return;
    end
end

end
